simulink model "Station_2_Handling_Processing"  (R2024a)
settings: Solver=VariableStepAuto  StartTime=0.0  StopTime=30  RelTol=1e-3
libraries: opcualib x1
settings Model: Creator=admin  LastModifiedBy=admin

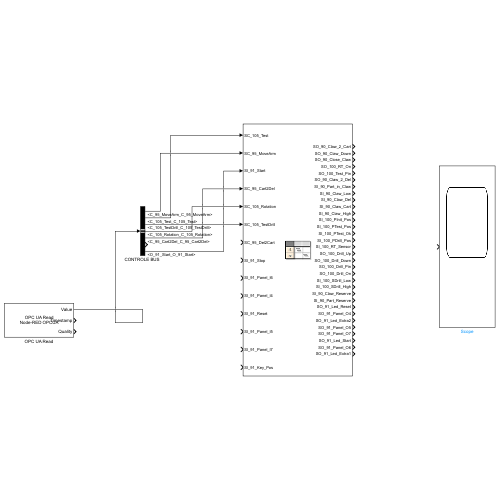
[thumbnail: Simulink's stored preview of the top-level diagram]
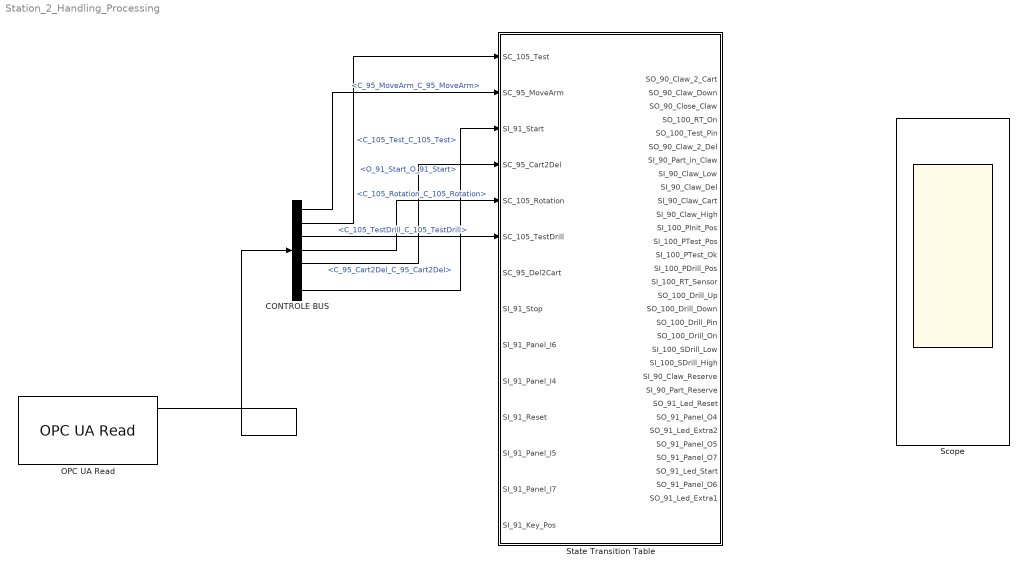
== system Station_2_Handling_Processing ==
  "CONTROLE BUS " : BusSelector  OutputSignals=C_95_MoveArm_C_95_MoveArm,C_105_Test_C_105_Test,C_105_TestDrill_C_105_TestDrill,C_105_Rotation_C_105_Rotation,C_95_Cart2Del_C_95_Cart2Del,C_95_Del2Cart_C_95_Del2Cart,O_91_Start_O_91_Start
  OPC UA Read : opcualib/OPC UA Read  SelectedServer=Node-RED OPCUA  ServerList=Node-RED OPCUA  NodeList={ '1', 'C_95_Cart2Del', '18', 'C_95_Cart2Del', '0'; '2', 'C_95_Del2Cart', '18', 'C_95_Del2Cart', '0'; '3', 'C_95_MoveArm', '18', 'C_95_MoveArm', '0'; '4', 'C_105_Test', '19', 'C_105_Test', '0'; '5', 'C_105_TestDrill', '19', 'C_105_TestDrill', '0'; '6', 'C_105_Rotation', '19', 'C_105_Rotation', '0'; '7', 'O_91_Start', '18', 'O_91_Start', '0'; '8', 'F_92_Claw_Down', '18', 'F_92_Claw_Down', '0'; '9', 'F_92_Close_Claw', '18', 'F_92_Close_Claw', '0'; '10', 'F_92_Claw_2_Del', '18', 'F_92_Claw_2_Del', '0'; '11', 'F_92_Claw_2_Cart', '18', 'F_92_Claw_2_Cart', '0'; '12', 'F_102_Drill_On', '19', 'F_102_Drill_On', '0'; '13', 'F_102_RT_On', '19', 'F_102_RT_On', '0'; '14', 'F_102_Drill_Down', '19', 'F_102_Drill_Down', '0'; '15', 'F_102_Drill_Up', '19', 'F_102_Drill_Up', '0'; '16', 'F_102_Drill_Pin', '19', 'F_102_Drill_Pin', '0'; '17', 'F_102_Test_Pin', '19', 'F_102_Test_Pin', '0'; '18', 'O_90_Claw_Del', '18', 'O_90_Claw_Del', '0'; '19', 'O_90_Claw_Cart', '18', 'O_90_Claw_Cart', '0'; '20', 'O_90_Claw_Low', '18', 'O_90_Claw_Low', '0'; '21', 'O_90_Claw_High', '18', 'O_90_Claw_High', '0'; '22', 'O_90_Part_in_Claw', '18', 'O_90_Part_in_Claw', '0'; '23', 'O_100_PInit_Pos', '19', 'O_100_PInit_Pos', '0'; '24', 'O_100_PDrill_Pos', '19', 'O_100_PDrill_Pos', '0'; '25', 'O_100_PTest_Pos', '19', 'O_100_PTest_Pos', '0'; '26', 'O_100_SDrill_High', '19', 'O_100_SDrill_High', '0'; '27', 'O_100_SDrill_Low', '19', 'O_100_SDrill_Low', '0'; '28', 'O_100_RT_Sensor', '19', 'O_100_RT_Sensor', '0'; '29', 'O_100_PTest_Ok', '19', 'O_100_PTest_Ok', '0' }  ShowQualityPort=on  ShowTimestampPort=on  ShowTimestampPortAs=Seconds since start  SampleTime=-1
  Scope : Scope
  State Transition Table : State Transition Table  TreatAsAtomicUnit=on
  wires:
  OPC UA Read/1 -> "CONTROLE BUS "/1
  "CONTROLE BUS "/1 -> State Transition Table/2(SC_95_MoveArm)  "<C_95_MoveArm_C_95_MoveArm>"
  "CONTROLE BUS "/2 -> State Transition Table/1(SC_105_Test)  "<C_105_Test_C_105_Test>"
  "CONTROLE BUS "/3 -> State Transition Table/6(SC_105_TestDrill)  "<C_105_TestDrill_C_105_TestDrill>"
  "CONTROLE BUS "/4 -> State Transition Table/5(SC_105_Rotation)  "<C_105_Rotation_C_105_Rotation>"
  "CONTROLE BUS "/5 -> State Transition Table/4(SC_95_Cart2Del)  "<C_95_Cart2Del_C_95_Cart2Del>"
  "CONTROLE BUS "/7 -> State Transition Table/3(SI_91_Start)  "<O_91_Start_O_91_Start>"

== stateflow chart Station_2_Handling_Processing/State Transition Table ==
  state state1
    SO_90_Claw_2_Cart=0;
    SO_90_Claw_2_Del=0;
    SO_90_Claw_Down=0;
    SO_90_Close_Claw=0;
    SO_100_RT_On=0;
    SO_100_Test_Pin=0;
    SI_90_Claw_Cart=1;
    SI_90_Claw_Low=0;
    SI_90_Claw_High=1;
    SI_90_Part_in_Claw=0;
    SI_90_Claw_Del=0;
    SI_100_PInit_Pos
    SI_100_PDrill_Pos=0;
    SI_100_PTest_Pos=0;
    SI_100_RT_Sensor=1;
    SI_100_PTest_Ok=0;
    SO_100_Drill_On=0;
    SO_100_Drill_Down=0;
    SO_100_Drill_Up=0;
    SO_100_Drill_Pin=0;
    SI_100_SDrill_High=1;
    SI_100_SDrill_Low=0;
    SI_90_Claw_Reserve=0;
    SI_90_Part_Reserve=0;
    SI_91_Stop;
    SI_91_Key_Pos;
    SI_91_Reset;
    SI_91_Panel_I4;
    SI_91_Panel_I5;
    SI_91_Panel_I6;
    SI_91_Panel_I7;
    SO_91_Led_Start=0;
    SO_91_Led_Reset=0;
    SO_91_Led_Extra1=0;
    SO_91_Led_Extra2=0;
    SO_91_Panel_O4=0;
    SO_91_Panel_O5=0;
    SO_91_Panel_O6=0;
    SO_91_Panel_O7=0;
  state claw_down
    SO_90_Claw_2_Cart=0;
    SO_90_Claw_2_Del=0;
    SO_90_Claw_Down=1;
    SO_90_Close_Claw=0;
    SO_100_RT_On=0;
    SO_100_Test_Pin=0;
    state claw_down_1
    (default) -> claw_down_1
    claw_down_1 -> (junction 672) : after(0.1,sec)
        | {SI_90_Claw_High=0;}
    (junction 672) -> claw_down_1
  state CLAW_UP
    SO_90_Claw_2_Cart=0;
    SO_90_Claw_2_Del=0;
    SO_90_Claw_Down=0;
    SO_90_Close_Claw=1;
    SO_100_RT_On=0;
    SO_100_Test_Pin=0;
    state CLAW_UP_1
    (default) -> CLAW_UP_1
    CLAW_UP_1 -> (junction 306) : after(1.8,sec)
        | {SI_90_Claw_Low=0;}
    (junction 306) -> CLAW_UP_1
  state claw_to_del
    SO_90_Claw_2_Cart=0;
    SO_90_Claw_2_Del=1;
    SO_90_Claw_Down=0;
    SO_90_Close_Claw=1;
    SO_100_RT_On=0;
    SO_100_Test_Pin=0;
    state claw_to_del_1
    (default) -> claw_to_del_1
    claw_to_del_1 -> (junction 302) : after(0.4,sec)
        | {SI_90_Claw_Cart=0;}
    (junction 302) -> claw_to_del_1
  state claw_down_at_cart
    SO_90_Claw_2_Cart=0;
    SO_90_Claw_2_Del=0;
    SO_90_Claw_Down=1;
    SO_90_Close_Claw=1;
    SO_100_RT_On=0;
    SO_100_Test_Pin=0;
    state claw_down_at_cart_1
    (default) -> claw_down_at_cart_1
    claw_down_at_cart_1 -> (junction 676) : after(0.1,sec)
        | {SI_90_Claw_High=0;}
    (junction 676) -> claw_down_at_cart_1
  state claw_up_at_del
    SO_90_Claw_2_Cart=0;
    SO_90_Claw_2_Del=0;
    SO_90_Claw_Down=0;
    SO_90_Close_Claw=0;
    SO_100_RT_On=0;
    SO_100_Test_Pin=0;
    state claw_up_at_del_1
    (default) -> claw_up_at_del_1
    claw_up_at_del_1 -> (junction 668) : after(0.25,sec)
        | {SI_90_Claw_Low=0;}
    (junction 668) -> claw_up_at_del_1
  state which_opperation
  state TEST_OPERATION_1
    SO_90_Claw_2_Del=0;
    SO_90_Claw_Down=0;
    SO_90_Close_Claw=0;
    SO_100_RT_On=1;
    SO_100_Test_Pin=0;
    state TEST_OPERATION_1_1
    state TEST_OPERATION_1_2
    state TEST_OPERATION_1_3
    state TEST_OPERATION_1_4
    TEST_OPERATION_1_4 -> (junction 404) : after(0.3,sec)
        | {SI_100_PDrill_Pos=0;
        | SI_100_PInit_Pos=0;
        | SI_100_PTest_Pos=0;}
    (default) -> TEST_OPERATION_1_1
    TEST_OPERATION_1_1 -> TEST_OPERATION_1_2 : after(0.1,sec)
        | {SI_100_RT_Sensor=0;
        | SI_100_PDrill_Pos=1;
        | SI_100_PInit_Pos=1;
        | SI_100_PTest_Pos=1;}
    TEST_OPERATION_1_2 -> TEST_OPERATION_1_3 : after(0.3,sec)
        | {SI_100_PDrill_Pos=0;
        | SI_100_PInit_Pos=0;
        | SI_100_PTest_Pos=0;}
    TEST_OPERATION_1_3 -> TEST_OPERATION_1_4 : after(0.5,sec)
        | {SI_100_PDrill_Pos=1;
        | SI_100_PInit_Pos=1;
        | SI_100_PTest_Pos=1;}
    (junction 404) -> TEST_OPERATION_1_4
  state TEST_OPERATION_2
    SO_90_Claw_2_Del=0;
    SO_90_Claw_Down=0;
    SO_90_Close_Claw=0;
    SO_100_RT_On=1;
    SO_100_Test_Pin=0;
    state TEST_OPERATION_2_1
    state TEST_OPERATION_2_2
    state TEST_OPERATION_2_3
    state TEST_OPERATION_2_4
    TEST_OPERATION_2_4 -> (junction 401) : after(0.3,sec)
        | {SI_100_PDrill_Pos=0;
        | SI_100_PInit_Pos=0;
        | SI_100_PTest_Pos=0;}
    (default) -> TEST_OPERATION_2_1
    TEST_OPERATION_2_1 -> TEST_OPERATION_2_2 : after(0.1,sec)
        | {SI_100_RT_Sensor=0;
        | SI_100_PDrill_Pos=1;
        | SI_100_PInit_Pos=1;
        | SI_100_PTest_Pos=1;}
    TEST_OPERATION_2_2 -> TEST_OPERATION_2_3 : after(0.3,sec)
        | {SI_100_PDrill_Pos=0;
        | SI_100_PInit_Pos=0;
        | SI_100_PTest_Pos=0;}
    TEST_OPERATION_2_3 -> TEST_OPERATION_2_4 : after(0.5,sec)
        | {SI_100_PDrill_Pos=1;
        | SI_100_PInit_Pos=1;
        | SI_100_PTest_Pos=1;}
    (junction 401) -> TEST_OPERATION_2_4
  state TEST_OPERATION_3
    SO_90_Claw_2_Del=0;
    SO_90_Claw_Down=0;
    SO_90_Close_Claw=0;
    SO_100_RT_On=1;
    SO_100_Test_Pin=0;
    state TEST_OPERATION_3_1
    state TEST_OPERATION_3_2
    state TEST_OPERATION_3_3
    state TEST_OPERATION_3_4
    (default) -> TEST_OPERATION_3_1
    TEST_OPERATION_3_1 -> TEST_OPERATION_3_2 : after(0.1,sec)
        | {SI_100_RT_Sensor=0;
        | SI_100_PDrill_Pos=1;
        | SI_100_PInit_Pos=1;
        | SI_100_PTest_Pos=1;}
    TEST_OPERATION_3_2 -> TEST_OPERATION_3_3 : after(0.3,sec)
        | {SI_100_PDrill_Pos=0;
        | SI_100_PInit_Pos=0;
        | SI_100_PTest_Pos=0;
        | SO_90_Claw_2_Cart=0;
        | SI_90_Claw_Cart=1;}
    TEST_OPERATION_3_3 -> TEST_OPERATION_3_4 : after(0.5,sec)
        | {SI_100_PDrill_Pos=1;
        | SI_100_PInit_Pos=1;
        | SI_100_PTest_Pos=1;}
    TEST_OPERATION_3_4 -> (junction 414) : after(0.3,sec)
        | {SI_100_PDrill_Pos=0;
        | SI_100_PInit_Pos=0;
        | SI_100_PTest_Pos=0;}
    (junction 414) -> TEST_OPERATION_3_4
  state TEST_OPERATION_4
    SO_90_Claw_2_Del=0;
    SO_90_Claw_Down=0;
    SO_90_Close_Claw=0;
    SO_100_RT_On=1;
    SO_100_Test_Pin=0;
    state TEST_OPERATION_4_1
    state TEST_OPERATION_4_2
    state TEST_OPERATION_4_3
    state TEST_OPERATION_4_4
    TEST_OPERATION_4_4 -> (junction 430) : after(0.3,sec)
        | {SI_100_PDrill_Pos=0;
        | SI_100_PInit_Pos=0;}
    (default) -> TEST_OPERATION_4_1
    TEST_OPERATION_4_1 -> TEST_OPERATION_4_2 : after(0.1,sec)
        | {SI_100_RT_Sensor=0;
        | SI_100_PDrill_Pos=1;
        | SI_100_PInit_Pos=1;
        | SI_100_PTest_Pos=1;}
    TEST_OPERATION_4_2 -> TEST_OPERATION_4_3 : after(0.3,sec)
        | {SI_100_PDrill_Pos=0;
        | SI_100_PInit_Pos=0;
        | SI_100_PTest_Pos=0;}
    TEST_OPERATION_4_3 -> TEST_OPERATION_4_4 : after(0.5,sec)
        | {SI_100_PDrill_Pos=1;
        | SI_100_PInit_Pos=1;
        | SI_100_PTest_Pos=1;}
    (junction 430) -> TEST_OPERATION_4_4
  state test_pin
    SO_90_Claw_2_Cart=0;
    SO_90_Claw_2_Del=0;
    SO_90_Claw_Down=0;
    SO_90_Close_Claw=0;
    SO_100_RT_On=0;
    SO_100_Test_Pin=1;
  state back_to_rt_1
    SO_90_Claw_2_Cart=0;
    SO_90_Claw_2_Del=0;
    SO_90_Claw_Down=0;
    SO_90_Close_Claw=0;
    SO_100_RT_On=1;
    SO_100_Test_Pin=0;
    state back_to_rt_1_1
    state back_to_rt_1_2
    state back_to_rt_1_3
    state back_to_rt_1_4
    back_to_rt_1_4 -> (junction 442) : after(0.3,sec)
        | {SI_100_PDrill_Pos=1;
        | SI_100_PInit_Pos=0;
        | SI_100_PTest_Pos=0;
        | SI_100_RT_Sensor=1;}
    (default) -> back_to_rt_1_1
    back_to_rt_1_1 -> back_to_rt_1_2 : after(0.1,sec)
        | {SI_100_PDrill_Pos=1;
        | SI_100_PInit_Pos=1;
        | SI_100_PTest_Pos=1;
        | SI_100_RT_Sensor=0;}
    back_to_rt_1_2 -> back_to_rt_1_3 : after(0.3,sec)
        | {SI_100_PDrill_Pos=0;
        | SI_100_PInit_Pos=0;
        | SI_100_PTest_Pos=0;}
    back_to_rt_1_3 -> back_to_rt_1_4 : after(0.5,sec)
        | {SI_100_PDrill_Pos=1;
        | SI_100_PInit_Pos=1;
        | SI_100_PTest_Pos=1;}
    (junction 442) -> back_to_rt_1_4
  state back_to_rt_2
    SO_90_Claw_2_Del=0;
    SO_90_Claw_Down=0;
    SO_90_Close_Claw=0;
    SO_100_RT_On=1;
    SO_100_Test_Pin=0;
    state back_to_rt_2_1
    state back_to_rt_2_2
    state back_to_rt_2_3
    state back_to_rt_2_4
    back_to_rt_2_4 -> (junction 451) : after(0.3,sec)
        | {SI_100_PDrill_Pos=0;
        | SI_100_PInit_Pos=1;
        | SI_100_PTest_Pos=0;
        | SI_100_RT_Sensor=1;}
    (default) -> back_to_rt_2_1
    back_to_rt_2_1 -> back_to_rt_2_2 : after(0.1,sec)
        | {SI_100_PDrill_Pos=1;
        | SI_100_PInit_Pos=1;
        | SI_100_PTest_Pos=1;
        | SI_100_RT_Sensor=0;}
    back_to_rt_2_2 -> back_to_rt_2_3 : after(0.3,sec)
        | {SI_100_PDrill_Pos=0;
        | SI_100_PInit_Pos=0;
        | SI_100_PTest_Pos=0;}
    back_to_rt_2_3 -> back_to_rt_2_4 : after(0.5,sec)
        | {SI_100_PDrill_Pos=1;
        | SI_100_PInit_Pos=1;
        | SI_100_PTest_Pos=1;}
    (junction 451) -> back_to_rt_2_4
  state ROTATION_OPERATION_1
    SO_90_Claw_2_Del=0;
    SO_90_Claw_Down=0;
    SO_90_Close_Claw=0;
    SO_100_RT_On=1;
    SO_100_Test_Pin=0;
    state ROTATION_OPERATION_1_1
    state ROTATION_OPERATION_1_2
    state ROTATION_OPERATION_1_3
    state ROTATION_OPERATION_1_4
    ROTATION_OPERATION_1.ROTATION_OPERATION_1_4 -> (junction 479) : after(0.3,sec)
        | {SI_100_PDrill_Pos=0;
        | SI_100_PInit_Pos=0;
        | SI_100_PTest_Pos=0;
        | SI_100_RT_Sensor=1;}
    (default) -> ROTATION_OPERATION_1_1
    ROTATION_OPERATION_1_1 -> ROTATION_OPERATION_1.ROTATION_OPERATION_1_2 : after(0.1,sec)
        | {SI_100_PDrill_Pos=1;
        | SI_100_PInit_Pos=1;
        | SI_100_PTest_Pos=1;
        | SI_100_RT_Sensor=0;}
    ROTATION_OPERATION_1.ROTATION_OPERATION_1_2 -> ROTATION_OPERATION_1.ROTATION_OPERATION_1_3 : after(0.3,sec)
        | {SI_100_PDrill_Pos=0;
        | SI_100_PInit_Pos=0;
        | SI_100_PTest_Pos=0;}
    ROTATION_OPERATION_1.ROTATION_OPERATION_1_3 -> ROTATION_OPERATION_1.ROTATION_OPERATION_1_4 : after(0.5,sec)
        | {SI_100_PDrill_Pos=1;
        | SI_100_PInit_Pos=1;
        | SI_100_PTest_Pos=1;}
    (junction 479) -> ROTATION_OPERATION_1.ROTATION_OPERATION_1_4
  state ROTATION_OPERATION_1_2
    SO_90_Claw_2_Del=0;
    SO_90_Claw_Down=0;
    SO_90_Close_Claw=0;
    SO_100_RT_On=1;
    SO_100_Test_Pin=0;
    state ROTATION_OPERATION_1_2_1
    state ROTATION_OPERATION_1_2_2
    state ROTATION_OPERATION_1_2_3
    state ROTATION_OPERATION_1_2_4
    ROTATION_OPERATION_1_2_4 -> (junction 491) : after(0.3,sec)
        | {SI_100_PDrill_Pos=0;
        | SI_100_PInit_Pos=0;
        | SI_100_PTest_Pos=0;
        | SI_100_RT_Sensor=1;}
    (default) -> ROTATION_OPERATION_1_2_1
    ROTATION_OPERATION_1_2_1 -> ROTATION_OPERATION_1_2_2 : after(0.1,sec)
        | {SI_100_PDrill_Pos=1;
        | SI_100_PInit_Pos=1;
        | SI_100_PTest_Pos=1;
        | SI_100_RT_Sensor=0;}
    ROTATION_OPERATION_1_2_2 -> ROTATION_OPERATION_1_2_3 : after(0.3,sec)
        | {SI_100_PDrill_Pos=0;
        | SI_100_PInit_Pos=0;
        | SI_100_PTest_Pos=0;}
    ROTATION_OPERATION_1_2_3 -> ROTATION_OPERATION_1_2_4 : after(0.5,sec)
        | {SI_100_PDrill_Pos=1;
        | SI_100_PInit_Pos=1;
        | SI_100_PTest_Pos=1;}
    (junction 491) -> ROTATION_OPERATION_1_2_4
  state ROTATION_OPERATION_1_3
    SO_90_Claw_2_Del=0;
    SO_90_Claw_Down=0;
    SO_90_Close_Claw=0;
    SO_100_RT_On=1;
    SO_100_Test_Pin=0;
    state ROTATION_OPERATION_1_3_1
    state ROTATION_OPERATION_1_3_2
    state ROTATION_OPERATION_1_3_3
    state ROTATION_OPERATION_1_3_4
    ROTATION_OPERATION_1_3_4 -> (junction 503) : after(0.3,sec)
        | {SI_100_PDrill_Pos=0;
        | SI_100_PInit_Pos=0;
        | SI_100_PTest_Pos=0;
        | SI_100_RT_Sensor=1;}
    (default) -> ROTATION_OPERATION_1_3_1
    ROTATION_OPERATION_1_3_1 -> ROTATION_OPERATION_1_3_2 : after(0.1,sec)
        | {SI_100_PDrill_Pos=1;
        | SI_100_PInit_Pos=1;
        | SI_100_PTest_Pos=1;
        | SI_100_RT_Sensor=0;}
    ROTATION_OPERATION_1_3_2 -> ROTATION_OPERATION_1_3_3 : after(0.3,sec)
        | {SI_100_PDrill_Pos=0;
        | SI_100_PInit_Pos=0;
        | SI_100_PTest_Pos=0;
        | SO_90_Claw_2_Cart=0;
        | SI_90_Claw_Cart=1;}
    ROTATION_OPERATION_1_3_3 -> ROTATION_OPERATION_1_3_4 : after(0.5,sec)
        | {SI_100_PDrill_Pos=1;
        | SI_100_PInit_Pos=1;
        | SI_100_PTest_Pos=1;}
    (junction 503) -> ROTATION_OPERATION_1_3_4
  state ROTATION_OPERATION_1_4
    SO_90_Claw_2_Del=0;
    SO_90_Claw_Down=0;
    SO_90_Close_Claw=0;
    SO_100_RT_On=1;
    SO_100_Test_Pin=0;
    state ROTATION_OPERATION_1_4_1
    state ROTATION_OPERATION_1_4_2
    state ROTATION_OPERATION_1_4_3
    state ROTATION_OPERATION_1_4_4
    ROTATION_OPERATION_1_4_4 -> (junction 515) : after(0.3,sec)
        | {SI_100_PDrill_Pos=0;
        | SI_100_PInit_Pos=0;
        | SI_100_PTest_Pos=1;
        | SI_100_RT_Sensor=1;}
    (default) -> ROTATION_OPERATION_1_4_1
    ROTATION_OPERATION_1_4_1 -> ROTATION_OPERATION_1_4_2 : after(0.1,sec)
        | {SI_100_PDrill_Pos=1;
        | SI_100_PInit_Pos=1;
        | SI_100_PTest_Pos=1;
        | SI_100_RT_Sensor=0;}
    ROTATION_OPERATION_1_4_2 -> ROTATION_OPERATION_1_4_3 : after(0.3,sec)
        | {SI_100_PDrill_Pos=0;
        | SI_100_PInit_Pos=0;
        | SI_100_PTest_Pos=0;}
    ROTATION_OPERATION_1_4_3 -> ROTATION_OPERATION_1_4_4 : after(0.5,sec)
        | {SI_100_PDrill_Pos=1;
        | SI_100_PInit_Pos=1;
        | SI_100_PTest_Pos=1;}
    (junction 515) -> ROTATION_OPERATION_1_4_4
  state ROTATION_OPERATION_1_5
    state ROTATION_OPERATION_1_5_1
    state ROTATION_OPERATION_1_5_2
    state ROTATION_OPERATION_1_5_3
    state ROTATION_OPERATION_1_5_4
    (default) -> ROTATION_OPERATION_1_5_1
    ROTATION_OPERATION_1_5_1 -> ROTATION_OPERATION_1_5_2 : after(0.1,sec)
        | {SI_100_PDrill_Pos=1;
        | SI_100_PInit_Pos=1;
        | SI_100_PTest_Pos=1;
        | SI_100_RT_Sensor=0;}
    ROTATION_OPERATION_1_5_2 -> ROTATION_OPERATION_1_5_3 : after(0.3,sec)
        | {SI_100_PDrill_Pos=0;
        | SI_100_PInit_Pos=0;
        | SI_100_PTest_Pos=0;
        | }
    ROTATION_OPERATION_1_5_3 -> ROTATION_OPERATION_1_5_4 : after(0.5,sec)
        | {SI_100_PDrill_Pos=1;
        | SI_100_PInit_Pos=1;
        | SI_100_PTest_Pos=1;}
    ROTATION_OPERATION_1_5_4 -> ROTATION_OPERATION_1_5_3 : after(0.3,sec)
        | {SI_100_PDrill_Pos=1;
        | SI_100_PInit_Pos=0;
        | SI_100_PTest_Pos=0;
        | SI_100_RT_Sensor=1;}
  state ROTATION_OPERATION_1_6
    SO_90_Claw_2_Del=0;
    SO_90_Claw_Down=0;
    SO_90_Close_Claw=0;
    SO_100_RT_On=1;
    SO_100_Test_Pin=0;
    state ROTATION_OPERATION_1_6_1
    state ROTATION_OPERATION_1_6_2
    state ROTATION_OPERATION_1_6_3
    state ROTATION_OPERATION_1_6_4
    ROTATION_OPERATION_1_6_4 -> (junction 537) : [after(0.3,sec)]
        | {SI_100_PDrill_Pos=0;
        | SI_100_PInit_Pos=1;
        | SI_100_PTest_Pos=0;
        | SI_100_RT_Sensor=1;}
    (default) -> ROTATION_OPERATION_1_6_1
    ROTATION_OPERATION_1_6_1 -> ROTATION_OPERATION_1_6_2 : after(0.1,sec)
        | {SI_100_PDrill_Pos=1;
        | SI_100_PInit_Pos=1;
        | SI_100_PTest_Pos=1;
        | SI_100_RT_Sensor=0;}
    ROTATION_OPERATION_1_6_2 -> ROTATION_OPERATION_1_6_3 : after(0.3,sec)
        | {SI_100_PDrill_Pos=0;
        | SI_100_PInit_Pos=0;
        | SI_100_PTest_Pos=0;
        | }
    ROTATION_OPERATION_1_6_3 -> ROTATION_OPERATION_1_6_4 : [after(0.5,sec)]
        | {SI_100_PDrill_Pos=1;
        | SI_100_PInit_Pos=1;
        | SI_100_PTest_Pos=1;}
    (junction 537) -> ROTATION_OPERATION_1_6_4
  state test_and_drill_rt
    SO_90_Claw_2_Cart=0;
    SO_90_Claw_2_Del=0;
    SO_90_Claw_Down=0;
    SO_90_Close_Claw=0;
    SO_100_RT_On=1;
    SO_100_Test_Pin=0;
    state test_and_drill_rt_1
    state test_and_drill_rt_2
    state test_and_drill_rt_3
    state test_and_drill_rt_4
    test_and_drill_rt_4 -> (junction 548) : after(0.3,sec)
        | {SI_100_PDrill_Pos=1;
        | SI_100_PInit_Pos=0;
        | SI_100_PTest_Pos=0;
        | SI_100_RT_Sensor=1;}
    (default) -> test_and_drill_rt_1
    test_and_drill_rt_1 -> test_and_drill_rt_2 : after(0.1,sec)
        | {SI_100_PDrill_Pos=1;
        | SI_100_PInit_Pos=1;
        | SI_100_PTest_Pos=1;
        | SI_100_RT_Sensor=0;}
    test_and_drill_rt_2 -> test_and_drill_rt_3 : after(0.3,sec)
        | {SI_100_PDrill_Pos=0;
        | SI_100_PInit_Pos=0;
        | SI_100_PTest_Pos=0;}
    test_and_drill_rt_3 -> test_and_drill_rt_4 : after(0.5,sec)
        | {SI_100_PDrill_Pos=1;
        | SI_100_PInit_Pos=1;
        | SI_100_PTest_Pos=1;}
    (junction 548) -> test_and_drill_rt_4
  state drill_down
    SO_90_Claw_2_Cart=0;
    SO_90_Claw_2_Del=0;
    SO_90_Claw_Down=0;
    SO_90_Close_Claw=0;
    SO_100_RT_On=0;
    SO_100_Test_Pin=0;
    SO_100_Drill_On=1;
    SO_100_Drill_Down=1;
    SO_100_Drill_Up=0;
    SO_100_Drill_Pin=1;
  state drill_up
    SO_90_Claw_2_Cart=0;
    SO_90_Claw_2_Del=0;
    SO_90_Claw_Down=0;
    SO_90_Close_Claw=0;
    SO_100_RT_On=0;
    SO_100_Test_Pin=0;
    SO_100_Drill_On=1;
    SO_100_Drill_Down=0;
    SO_100_Drill_Up=1;
    SO_100_Drill_Pin=1;
  state last_rt
    SO_90_Claw_2_Cart=0;
    SO_90_Claw_2_Del=0;
    SO_90_Claw_Down=0;
    SO_90_Close_Claw=0;
    SO_100_RT_On=1;
    SO_100_Test_Pin=0;
    SO_100_Drill_On=0;
    SO_100_Drill_Down=0;
    SO_100_Drill_Up=0;
    SO_100_Drill_Pin=0;
    state last_rt_1
    state last_rt_2
    state last_rt_3
    state last_rt_4
    last_rt_4 -> (junction 553) : after(0.3,sec)
        | {SI_100_PDrill_Pos=0;
        | SI_100_PInit_Pos=1;
        | SI_100_PTest_Pos=0;
        | SI_100_RT_Sensor=1;}
    (default) -> last_rt_1
    last_rt_1 -> last_rt_2 : after(0.1,sec)
        | {SI_100_PDrill_Pos=1;
        | SI_100_PInit_Pos=1;
        | SI_100_PTest_Pos=1;
        | SI_100_RT_Sensor=0;}
    last_rt_2 -> last_rt_3 : after(0.3,sec)
        | {SI_100_PDrill_Pos=0;
        | SI_100_PInit_Pos=0;
        | SI_100_PTest_Pos=0;}
    last_rt_3 -> last_rt_4 : after(0.5,sec)
        | {SI_100_PDrill_Pos=1;
        | SI_100_PInit_Pos=1;
        | SI_100_PTest_Pos=1;}
    (junction 553) -> last_rt_4
  state reverse_operation
    SO_90_Claw_2_Cart=0;
    SO_90_Claw_2_Del=1;
    SO_90_Claw_Down=0;
    SO_90_Close_Claw=0;
    state reverse_operation_1
    (default) -> reverse_operation_1
    reverse_operation_1 -> (junction 602) : after(0.4,sec)
        | {SI_90_Claw_Cart=0;}
    (junction 602) -> reverse_operation_1
  state claw_down_r
    SO_90_Claw_2_Cart=0;
    SO_90_Claw_2_Del=0;
    SO_90_Claw_Down=1;
    SO_90_Close_Claw=0;
    state claw_down_r_1
    (default) -> claw_down_r_1
    claw_down_r_1 -> (junction 680) : after(0.1,sec)
        | {SI_90_Claw_High=0;}
    (junction 680) -> claw_down_r_1
  state claw_up_r
    SO_90_Claw_2_Cart=0;
    SO_90_Claw_2_Del=0;
    SO_90_Claw_Down=0;
    SO_90_Close_Claw=1;
    state claw_up_r_1
    (default) -> claw_up_r_1
    claw_up_r_1 -> (junction 606) : after(0.25,sec)
        | {
        | SI_90_Claw_Low=0;}
    (junction 606) -> claw_up_r_1
  state claw_2_cart_r
    SO_90_Claw_2_Cart=1;
    SO_90_Claw_2_Del=0;
    SO_90_Claw_Down=0;
    SO_90_Close_Claw=1;
    state claw_2_cart_r_1
    (default) -> claw_2_cart_r_1
    claw_2_cart_r_1 -> (junction 610) : after(0.4,sec)
        | {SI_90_Claw_Del=0;}
    (junction 610) -> claw_2_cart_r_1
  state claw_down_r_2
    SO_90_Claw_2_Cart=0;
    SO_90_Claw_2_Del=0;
    SO_90_Claw_Down=1;
    SO_90_Close_Claw=1;
  state state2
    SO_90_Claw_2_Cart=0;
    SO_90_Claw_2_Del=0;
    SO_90_Claw_Down=0;
    SO_90_Close_Claw=0;
    state state2_1
    (default) -> state2_1
    state2_1 -> (junction 614) : after(0.25,sec)
        | {SI_90_Claw_Low=0;}
    (junction 614) -> state2_1
  state CLAW_DOWN_RES1
    SO_90_Claw_2_Cart=0;
    SO_90_Claw_2_Del=0;
    SO_90_Claw_Down=1;
    SO_90_Close_Claw=0;
    state CLAW_DOWN_RES1_1
    (default) -> CLAW_DOWN_RES1_1
    CLAW_DOWN_RES1_1 -> (junction 699) : after(0.1,sec)
        | {SI_90_Claw_High=0;}
    (junction 699) -> CLAW_DOWN_RES1_1
  state CLAW_UP_RES
    SO_90_Claw_2_Cart=0;
    SO_90_Claw_2_Del=0;
    SO_90_Claw_Down=0;
    SO_90_Close_Claw=1;
    state CLAW_UP_RES_1
    (default) -> CLAW_UP_RES_1
    CLAW_UP_RES_1 -> (junction 630) : after(1.2,sec)
        | {SI_90_Claw_Low=0;}
    (junction 630) -> CLAW_UP_RES_1
  state TO_RESERVE
    SO_90_Claw_2_Cart=0;
    SO_90_Claw_2_Del=1;
    SO_90_Claw_Down=0;
    SO_90_Close_Claw=1;
    state TO_RESERVE_1
    (default) -> TO_RESERVE_1
    TO_RESERVE_1 -> (junction 684) : after(0.1,sec)
        | {SI_90_Claw_Cart=0;}
    (junction 684) -> TO_RESERVE_1
  state claw_down_at_res
    SO_90_Claw_2_Cart=0;
    SO_90_Claw_2_Del=0;
    SO_90_Claw_Down=1;
    SO_90_Close_Claw=1;
    state claw_down_at_res_1
    (default) -> claw_down_at_res_1
    claw_down_at_res_1 -> (junction 688) : after(0.15,sec)
        | {SI_90_Claw_Reserve=0;}
    (junction 688) -> claw_down_at_res_1
  state claw_UP_at_res
    SO_90_Claw_2_Cart=0;
    SO_90_Claw_2_Del=0;
    SO_90_Claw_Down=0;
    SO_90_Close_Claw=0;
    state claw_UP_at_res_1
    (default) -> claw_UP_at_res_1
    claw_UP_at_res_1 -> (junction 644) : after(0.25,sec)
        | {SI_90_Claw_Low=0;}
    (junction 644) -> claw_UP_at_res_1
  state BACK_TO_CART
    SO_90_Claw_2_Cart=1;
    SO_90_Claw_2_Del=0;
    SO_90_Claw_Down=0;
    SO_90_Close_Claw=0;
  (default) -> state1
  (junction 365) -> state1
  state1 -> (junction 567) [order 2] : [((SI_91_Start==1 || SC_95_MoveArm==1 )&&( SC_95_Del2Cart==1 )) && SI_100_PInit_Pos==1 ]
  (junction 367) -> (junction 365)
  (junction 567) -> (junction 565)
  state1 -> (junction 598) [order 3] : [((SI_91_Start==1 || SC_95_MoveArm==1 )&&( SC_95_Cart2Del==1 )) && SI_100_PInit_Pos==1 ]
  (junction 598) -> (junction 596)
  state1 -> claw_down [order 1] : [(SI_91_Start==1 || SC_95_MoveArm==1 )&&( SC_95_Cart2Del==1 )  ]
  claw_down -> CLAW_UP : after(0.65,sec)
      | {SI_90_Claw_Low=1;
      | SI_90_Part_in_Claw=1;}
  CLAW_UP -> claw_to_del : after(2.4,sec)
      | {SI_90_Claw_High=1;}
  claw_to_del -> claw_down_at_cart : after(3.4,sec)
      | {SI_90_Claw_Del=1;}
  claw_down_at_cart -> claw_up_at_del : after(0.65,sec)
      | {SI_90_Claw_Low=1;
      | SI_90_Part_in_Claw=0;
      | SI_100_PInit_Pos=1; }
  claw_up_at_del -> which_opperation : after(0.8,sec)
      | {SI_90_Claw_High=1;}
  which_opperation -> (junction 54) [order 2] : [SC_105_Rotation==1]
      | {SI_90_Claw_Del=0;
      | SI_100_PDrill_Pos=1;
      | SI_100_PTest_Pos=1;
      | SI_100_RT_Sensor=1;
      | SO_90_Claw_2_Cart=1;}
  (junction 54) -> (junction 52)
  which_opperation -> TEST_OPERATION_1 [order 1] : [SC_105_Test==1]
      | {SI_90_Claw_Del=0;
      | SI_100_PDrill_Pos=0;
      | SI_100_PTest_Pos=0;
      | SI_100_RT_Sensor=0;
      | SO_90_Claw_2_Cart=1;}
  which_opperation -> TEST_OPERATION_1 [order 3] : [SC_105_TestDrill==1]
      | {SI_90_Claw_Del=0;
      | SO_90_Claw_2_Cart=1;}
  TEST_OPERATION_1 -> TEST_OPERATION_2 : after(1.2,sec)
      | {SI_100_RT_Sensor=1;}
  TEST_OPERATION_2 -> TEST_OPERATION_3 : after(1.2,sec)
      | {SI_100_RT_Sensor=1;}
  TEST_OPERATION_3 -> TEST_OPERATION_4 : after(1.2,sec)
      | {SI_100_RT_Sensor=1;}
  TEST_OPERATION_4 -> test_pin : after(1.2,sec)
      | {SI_100_PDrill_Pos=0;
      | SI_100_PInit_Pos=0;
      | SI_100_RT_Sensor=1;
      | SI_100_PTest_Ok=1;}
  test_pin -> (junction 239) [order 2] : [after(1.2,sec)&& SC_105_TestDrill==1]
      | {SI_100_PTest_Ok=0;}
  (junction 239) -> (junction 237)
  test_pin -> back_to_rt_1 [order 1] : [after(1.2,sec)&& SC_105_TestDrill==0]
      | {SI_100_PTest_Ok=0;}
  back_to_rt_1 -> back_to_rt_2 : after(1.2,sec)
      | {SI_100_PInit_Pos=1;
      | SI_100_PDrill_Pos=0;
      | SI_100_PTest_Pos=0;
      | SI_100_RT_Sensor=1;}
  back_to_rt_2 -> (junction 367) : after(1.2,sec)
  (junction 561) -> (junction 367)
  (junction 52) -> ROTATION_OPERATION_1
  ROTATION_OPERATION_1 -> ROTATION_OPERATION_1_2 : after(1.2,sec)
  ROTATION_OPERATION_1_2 -> ROTATION_OPERATION_1_3 : after(1.2,sec)
  ROTATION_OPERATION_1_3 -> ROTATION_OPERATION_1_4 : after(1.2,sec)
  ROTATION_OPERATION_1_4 -> ROTATION_OPERATION_1_5 : after(1.2,sec)
  ROTATION_OPERATION_1_5 -> ROTATION_OPERATION_1_6 : after(1.2,sec)
  ROTATION_OPERATION_1_6 -> (junction 561) : after(1.2,sec)
  (junction 558) -> (junction 561)
  (junction 237) -> test_and_drill_rt
  test_and_drill_rt -> drill_down : after(1.2,sec)
  drill_down -> drill_up : after(1.8,sec)
      | {SI_100_PTest_Pos=0;
      | SI_100_PDrill_Pos=0;
      | SI_100_PInit_Pos=0;
      | SI_100_RT_Sensor=0;
      | SI_100_SDrill_Low=0;
      | SI_100_SDrill_High=1;}
  drill_up -> last_rt : after(0.6,sec)
      | {SI_100_PDrill_Pos=0;
      | SI_100_PInit_Pos=0;
      | SI_100_PTest_Pos=0;
      | SI_100_RT_Sensor=0;}
  last_rt -> (junction 558) : after(1.2,sec)
  (junction 592) -> (junction 558)
  (junction 565) -> reverse_operation
  reverse_operation -> claw_down_r : after(3.55,sec)
      | {SI_90_Claw_Del=1;}
  claw_down_r -> claw_up_r : after(0.65,sec)
      | {SI_90_Claw_Low=1;
      | SI_90_Part_in_Claw=1;}
  claw_up_r -> claw_2_cart_r : after(0.8,sec)
      | {SI_90_Claw_High=1;}
  claw_2_cart_r -> claw_down_r_2 : after(2.5,sec)
      | {SI_90_Claw_Cart=1;
      | SI_90_Claw_High=0;}
  claw_down_r_2 -> state2 : after(0.6,sec)
      | {SI_90_Claw_Low=1;
      | SI_90_Part_in_Claw=0;}
  state2 -> (junction 592) : after(0.8,sec)
  (junction 692) -> (junction 592)
  (junction 596) -> CLAW_DOWN_RES1
  CLAW_DOWN_RES1 -> CLAW_UP_RES : after(0.65,sec)
      | {SI_90_Claw_Low=1;
      | SI_90_Part_in_Claw=1;}
  CLAW_UP_RES -> TO_RESERVE : after(1.8,sec)
      |
      | {SI_90_Claw_High=1;}
  TO_RESERVE -> claw_down_at_res : after(1.2,sec)
      | {SI_90_Claw_Reserve=1;
      | SI_90_Claw_High=0;}
  claw_down_at_res -> claw_UP_at_res : after(0.65,sec)
      | {SI_90_Claw_Low=1;
      | SI_90_Part_in_Claw=0;
      | SI_90_Part_Reserve=1;}
  claw_UP_at_res -> BACK_TO_CART : after(0.8,sec)
      |
      | {SI_90_Claw_High=1;
      | }
  BACK_TO_CART -> (junction 692) : after(1.1,sec)
      | {SI_90_Claw_Cart=1;}
  data: SC_105_Test input; SC_95_MoveArm input; SI_91_Start input; SC_95_Cart2Del input; SC_105_Rotation input; SO_90_Claw_2_Cart output; SO_90_Claw_Down output; SO_90_Close_Claw output; SO_100_RT_On output; SO_100_Test_Pin output; SO_90_Claw_2_Del output; SI_90_Part_in_Claw output; SI_90_Claw_Low output; SI_90_Claw_Del output; SI_90_Claw_Cart output; SI_90_Claw_High output; SI_100_PInit_Pos output; SI_100_PTest_Pos output; SI_100_PTest_Ok output; SI_100_PDrill_Pos output; SI_100_RT_Sensor output; SC_105_TestDrill input; SO_100_Drill_Up output; SO_100_Drill_Down output; SO_100_Drill_Pin output; SO_100_Drill_On output; SI_100_SDrill_Low output; SI_100_SDrill_High output; SC_95_Del2Cart input; SI_90_Claw_Reserve output; SI_90_Part_Reserve output; SI_91_Stop input; SI_91_Panel_I6 input; SI_91_Panel_I4 input; SI_91_Reset input; SI_91_Panel_I5 input; SI_91_Panel_I7 input; SI_91_Key_Pos input; SO_91_Led_Reset output; SO_91_Panel_O4 output; SO_91_Led_Extra2 output; SO_91_Panel_O5 output; SO_91_Panel_O7 output; SO_91_Led_Start output; SO_91_Panel_O6 output; SO_91_Led_Extra1 output
